simulink model "control_sim"  (R2019b)
settings: Solver=VariableStepAuto  StartTime=0.0  StopTime=T  MaxStep=t_step  RelTol=1e-3
values from neighbouring files (symbols this model uses):
  H_tr = H_tr(1:2,:)    [main.m]
  Pe0 = zeros([nx nx])    [main.m]
  T = times(end)    [DataStore.m]    (also in getTrajectoryFromPoints.m = size(x1, 2)*t_step)
  x0_nom = traj_simple.x.data(1:nx,1,1)    [main.m]
undefined symbols (not defined in the file or in its folder): dis_amp, variance
settings Model: Creator=Lenovo A9 Ssd  LastModifiedBy=Lenovo A9 Ssd

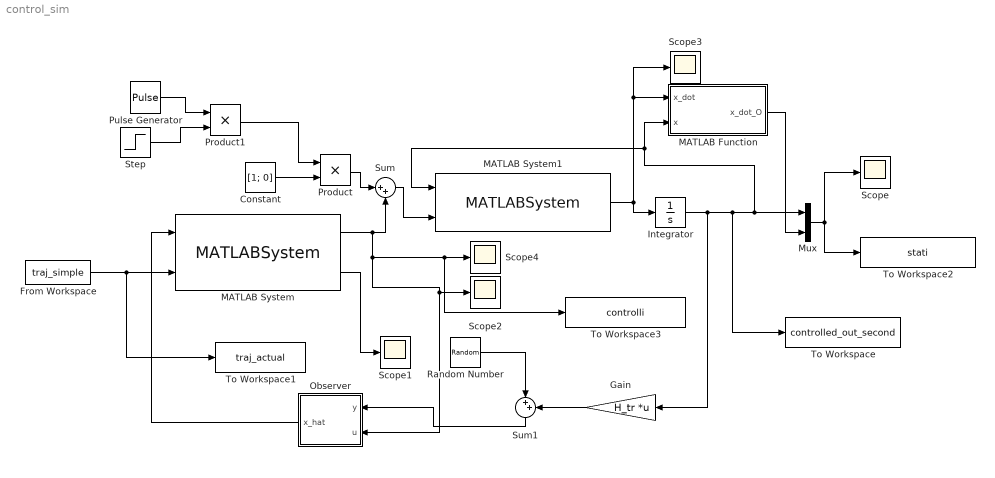
== system control_sim ==
  Constant : Constant  Value=[1; 0]
  From Workspace : FromWorkspace  VariableName=traj_simple  OutDataTypeStr=Bus: traj_bus  SampleTime=0
  Gain : Gain  Gain=H_tr  Multiplication=Matrix(K*u)
  Integrator : Integrator  InitialCondition=x0_nom
  MATLAB Function : MATLAB Function  TreatAsAtomicUnit=on
  MATLAB System : MATLABSystem  System=simplecontroller  weights=weights  model_params=model_params  H_tr=H_tr  threshold=0.5  x0=x0_nom  u0=u0  SimulateUsing=Interpreted execution
      mask Type: simplecontroller
      mask Display:
      | disp('simplecontroller');
      | port_label('input',1,'x');
      | port_label('input',2,'traj');
      | port_label('output',1,'u');
      | port_label('output',2,'closest');
  MATLAB System1 : MATLABSystem  System=ModelSys  model_params=model_params  SimulateUsing=Interpreted execution
      mask Type: ModelSys
      mask Display:
      | disp('ModelSys');
      | port_label('input',1,'x');
      | port_label('input',2,'u');
      | port_label('output',1,'x_dot');
  Mux : Mux  Inputs=2
  Observer : Subsystem
  Product : Product
  Product1 : Product
  Pulse Generator : DiscretePulseGenerator  PulseType=Time based  Amplitude=dis_amp  Period=T/1.99
  Random Number : RandomNumber  Mean=[0, 0]  Variance=variance
  Scope{,1..4} (5 alike) : Scope
  Step : Step  Time=T/1.99  SampleTime=0
  Sum : Sum  Inputs=|++
  Sum1 : Sum  Inputs=|++
  To Workspace : ToWorkspace  VariableName=controlled_out_second  SaveFormat=Timeseries  SampleTime=-1
  To Workspace1 : ToWorkspace  VariableName=traj_actual  SaveFormat=Timeseries  SampleTime=-1
  To Workspace2 : ToWorkspace  VariableName=stati  SaveFormat=Timeseries  SampleTime=-1
  To Workspace3 : ToWorkspace  VariableName=controlli  SaveFormat=Timeseries  SampleTime=-1
  wires:
  MATLAB System1/1 -> Scope3/1, MATLAB Function/1(x_dot), Integrator/1
  Integrator/1 -> Gain/1, MATLAB System1/1, MATLAB Function/2(x), Mux/1, To Workspace/1
  From Workspace/1 -> To Workspace1/1, MATLAB System/2
  MATLAB System/2 -> Scope1/1
  Gain/1 -> Sum1/2
  MATLAB Function/1(x_dot_O) -> Mux/2
  Mux/1 -> Scope/1, To Workspace2/1
  Observer/1(x_hat) -> MATLAB System/1
  MATLAB System/1 -> Sum/2, To Workspace3/1, Scope4/1, Observer/2(u), Scope2/1
  Random Number/1 -> Sum1/1
  Sum1/1 -> Observer/1(y)
  Constant/1 -> Product/2
  Product/1 -> Sum/1
  Sum/1 -> MATLAB System1/2
  Pulse Generator/1 -> Product1/1
  Step/1 -> Product1/2
  Product1/1 -> Product/1

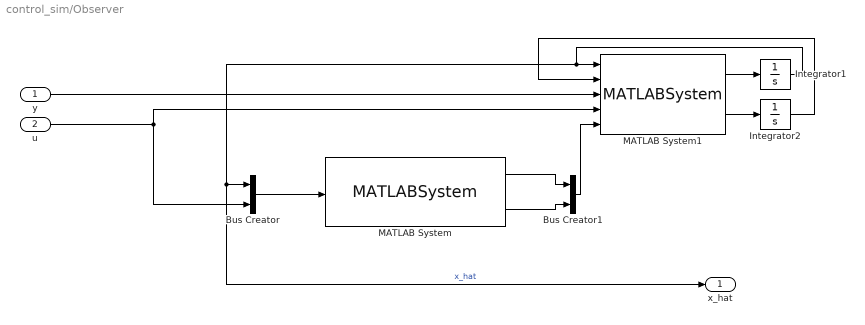
== system control_sim/Observer ==
  y : Inport
  u : Inport  Port=2
  Bus Creator : BusCreator  Inputs=2  OutDataTypeStr=Bus: traj_bus
  Bus Creator1 : BusCreator  Inputs=2  OutDataTypeStr=Bus: lin_mat_bus
  Integrator1 : Integrator  InitialCondition=x0_nom
  Integrator2 : Integrator  InitialCondition=Pe0
  MATLAB System : MATLABSystem  System=Linearizer  model_params=model_params  SimulateUsing=Interpreted execution
      mask Type: Linearizer
      mask Display:
      | disp('Linearizer');
      | port_label('input',1,'traj');
      | port_label('output',1,'F');
      | port_label('output',2,'G');
  MATLAB System1 : MATLABSystem  System=Observer  weights_obs=weights_obs  model_params=model_params  H_tr=H_tr  SimulateUsing=Interpreted execution
      mask Type: Observer
      mask Display:
      | disp('Observer');
      | port_label('input',1,'x_hat');
      | port_label('input',2,'Pe');
      | port_label('input',3,'y');
      | port_label('input',4,'u');
      | port_label('input',5,'lin_params');
      | port_label('output',1,'x_hat_dot');
      | port_label('output',2,'Pe_dot');
  x_hat : Outport
  wires:
  MATLAB System/1 -> Bus Creator1/1
  MATLAB System1/1 -> Integrator1/1
  MATLAB System/2 -> Bus Creator1/2
  u/1 -> MATLAB System1/4, Bus Creator/2
  Integrator1/1 -> MATLAB System1/1, x_hat/1, Bus Creator/1  "x_hat"
  Bus Creator/1 -> MATLAB System/1
  Integrator2/1 -> MATLAB System1/2
  Bus Creator1/1 -> MATLAB System1/5
  MATLAB System1/2 -> Integrator2/1
  y/1 -> MATLAB System1/3

== matlab function control_sim/MATLAB Function ==
  data: x_dot input; x_dot_O output; x input
function x_dot_O = fcn(x_dot, x)
    psi = x(3);
    R_O_W = [cos(psi), - sin(psi);
             sin(psi), cos(psi)]';
    x_dot_O = R_O_W *x_dot(1:2, :);
